simulink model "simulation"  (R2018b)
settings: Solver=VariableStepAuto  StartTime=0.0  StopTime=20  RelTol=1e-3
values from neighbouring files (symbols this model uses):
  f = 1    [parameters.m]
  k = 9    [parameters.m]
  lambda0 = 1    [parameters.m]
  M = 10    [parameters.m]
  p0 = 1    [parameters.m]
settings Model: Creator=cale  LastModifiedBy=cale

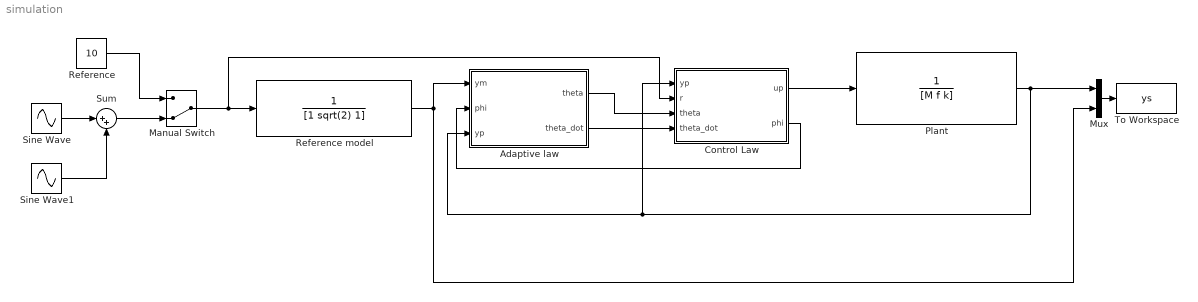
== system simulation ==
  Adaptive law : Subsystem
  Control Law : Subsystem
  Manual Switch : ManualSwitch  CurrentSetting=0
  Mux : Mux  Inputs=2
  Plant : TransferFcn  Denominator=[M f k]  ContinuousStateAttributes='y_p'
  Reference : Constant  Value=10
  Reference model : TransferFcn  Denominator=[1 sqrt(2) 1]  ContinuousStateAttributes='y_m'
  Sine Wave : Sin  Amplitude=2  Frequency=3  SampleTime=0
  Sine Wave1 : Sin  Amplitude=5  SampleTime=0
  Sum : Sum  Inputs=|++
  To Workspace : ToWorkspace  VariableName=ys  SaveFormat=Timeseries  SampleTime=-1
  wires:
  Control Law/1(up) -> Plant/1
  Plant/1 -> Mux/1, Adaptive law/3(yp), Control Law/1(yp)
  Reference model/1 -> Mux/2, Adaptive law/1(ym)
  Control Law/2(phi) -> Adaptive law/2(phi)
  Adaptive law/1(theta) -> Control Law/3(theta)
  Adaptive law/2(theta_dot) -> Control Law/4(theta_dot)
  Reference/1 -> Manual Switch/1
  Manual Switch/1 -> Control Law/2(r), Reference model/1
  Sum/1 -> Manual Switch/2
  Sine Wave/1 -> Sum/1
  Sine Wave1/1 -> Sum/2
  Mux/1 -> To Workspace/1

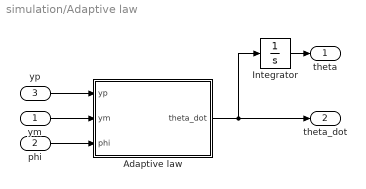
== system simulation/Adaptive law ==
  ym : Inport
  phi : Inport  Port=2
  yp : Inport  Port=3
  Adaptive law : MATLAB Function  TreatAsAtomicUnit=on
  Integrator : Integrator
  theta : Outport
  theta_dot : Outport  Port=2
  wires:
  yp/1 -> Adaptive law/1(yp)
  phi/1 -> Adaptive law/3(phi)
  Adaptive law/1(theta_dot) -> theta_dot/1, Integrator/1
  ym/1 -> Adaptive law/2(ym)
  Integrator/1 -> theta/1

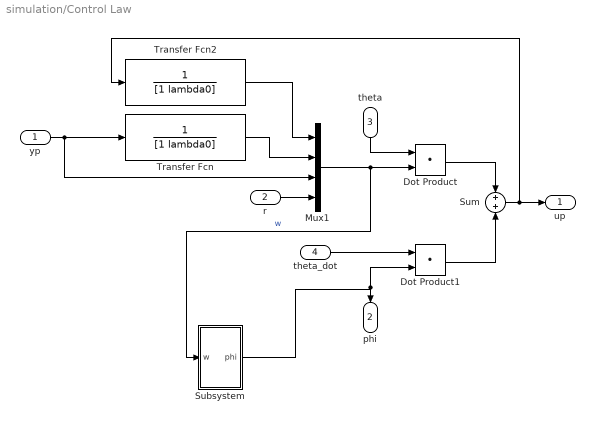
== system simulation/Control Law ==
  yp : Inport
  r : Inport  Port=2
  theta : Inport  Port=3
  theta_dot : Inport  Port=4
  Dot Product : DotProduct  InputSameDT=on  OutDataTypeStr=Inherit: Inherit via internal rule
  Dot Product1 : DotProduct  InputSameDT=on  OutDataTypeStr=Inherit: Inherit via internal rule
  Mux1 : Mux
  Subsystem : Subsystem
  Sum : Sum  Inputs=+|+
  Transfer Fcn : TransferFcn  Denominator=[1 lambda0]
  Transfer Fcn2 : TransferFcn  Denominator=[1 lambda0]
  up : Outport
  phi : Outport  Port=2
  wires:
  yp/1 -> Mux1/3, Transfer Fcn/1
  theta/1 -> Dot Product/1
  Mux1/1 -> Subsystem/1(w), Dot Product/2  "w"
  Dot Product/1 -> Sum/1
  theta_dot/1 -> Dot Product1/1
  Subsystem/1(phi) -> Dot Product1/2, phi/1
  Dot Product1/1 -> Sum/2
  Sum/1 -> up/1, Transfer Fcn2/1
  r/1 -> Mux1/4
  Transfer Fcn2/1 -> Mux1/1
  Transfer Fcn/1 -> Mux1/2

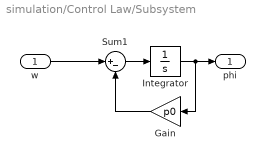
== system simulation/Control Law/Subsystem ==
  w : Inport
  Gain : Gain  Gain=p0
  Integrator : Integrator
  Sum1 : Sum  Inputs=|+-
  phi : Outport
  wires:
  Integrator/1 -> phi/1, Gain/1
  w/1 -> Sum1/1
  Sum1/1 -> Integrator/1
  Gain/1 -> Sum1/2

== matlab function simulation/Adaptive law/Adaptive law ==
  data: yp input; theta_dot output; ym input; phi input
function theta_dot  = fcn(yp, ym, phi)

Gamma = diag([1,1,1,1]);

e1 = yp - ym;

theta_dot = -Gamma*e1*phi;
